simulink model "robotarm_A2_breach"  (R2018b)
settings: Solver=FixedStepAuto  StartTime=0.0  StopTime=tspan(end)  RelTol=1e-3  AbsTol=1e-6
undefined symbols (not defined in the file): options
libraries: neural x132, simulink x2
(part 2 of 6)

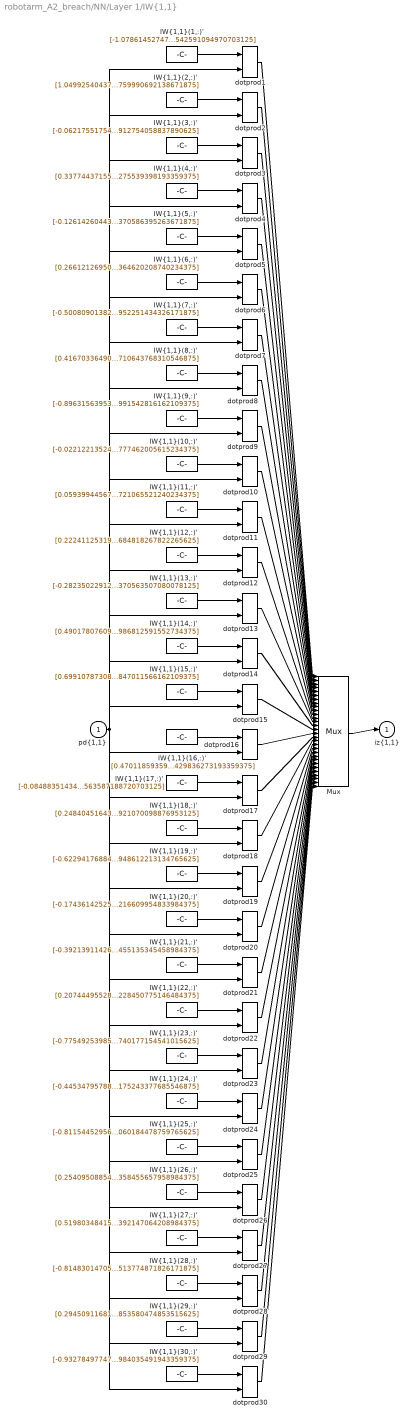
== system robotarm_A2_breach/NN/Layer 1/IW{1,1} ==
  "pd{1,1}" : Inport  PortDimensions=10
      mask Display: e = 0.06;c1 = [120 230 180]/255;c2 = ([120 230 180]+0)/(256+128);c3 = ([120 230 180]+128)/(256+128);patch([0 1 1 0],[0 0 1 1],c1);patch([0 1 1 1-e 1-e 0+e],[0 0 1 1-e 0+e 0+e],c2);patch([0 0 1 1-e 0+e 0+e],[0 1 1 1-e 1-e 0+e],c3);plot([0 1 1 0 0],[0 0 1 1 0]);
  "IW{1,1}(1,:)'" : Constant  Value=[-1.0786145274703653473835629483801312744617462158203125;0.77264081663859851545339552103541791439056396484375;0.93405870513662414555966506668482907116413116455078125;-0.012284087004165382406295492501158150844275951385498046875;-0.07882050130441907442868654243284254334867000579833984375;0.449587152172945092587497128988616168498992919921875;0.2441305252532121328190584108597249723970890045166015625;0.46267379659151774973224746645428240299224853515625;0.31528848398154940557702730075106956064701080322265625;0.592770821508250111975257823360152542591094970703125]
      mask Display: e = 0.06;c1 = [120 150 230]/255;c2 = ([120 150 230]+0)/383;c3 = ([120 150 230]+128)/383;patch([0 1 1 0],[0 0 1 1],c1);patch([0 1 1 1-e 1-e 0+e],[0 0 1 1-e 0+e 0+e],c2);patch([0 0 1 1-e 0+e 0+e],[0 1 1 1-e 1-e 0+e],c3);plot([0 1 1 0 0],[0 0 1 1 0]);disp('Weights');
  "IW{1,1}(10,:)'" : Constant  Value=[-0.02212213524676130693702447160831070505082607269287109375;0.70448840071230034443061640558880753815174102783203125;-0.38943718547013428388225975140812806785106658935546875;0.060339806407884423455900702037979499436914920806884765625;0.97898368743937858038606236732448451220989227294921875;-0.8612083675280104433369388061692006886005401611328125;0.16399922308413772409352304748608730733394622802734375;0.2354951023310313529268711363329202868044376373291015625;0.57616029420315928444296105226385407149791717529296875;-0.31121188855659320804392109494074247777462005615234375]
      mask Display: e = 0.06;c1 = [120 150 230]/255;c2 = ([120 150 230]+0)/383;c3 = ([120 150 230]+128)/383;patch([0 1 1 0],[0 0 1 1],c1);patch([0 1 1 1-e 1-e 0+e],[0 0 1 1-e 0+e 0+e],c2);patch([0 0 1 1-e 0+e 0+e],[0 1 1 1-e 1-e 0+e],c3);plot([0 1 1 0 0],[0 0 1 1 0]);disp('Weights');
  "IW{1,1}(11,:)'" : Constant  Value=[0.05939944567701915811852586557506583631038665771484375;-0.6082056891321736546984766391688026487827301025390625;1.03721893251289554171989948372356593608856201171875;0.4534212907984009888195942039601504802703857421875;-0.648457002097055035250150467618368566036224365234375;0.74638444669292958177919672380085103213787078857421875;-0.7295656890584074627525978939956985414028167724609375;0.306888274274469463609449348950874991714954376220703125;0.452997445555755662294217245289473794400691986083984375;0.62071804133911834266967844087048433721065521240234375]
      mask Display: e = 0.06;c1 = [120 150 230]/255;c2 = ([120 150 230]+0)/383;c3 = ([120 150 230]+128)/383;patch([0 1 1 0],[0 0 1 1],c1);patch([0 1 1 1-e 1-e 0+e],[0 0 1 1-e 0+e 0+e],c2);patch([0 0 1 1-e 0+e 0+e],[0 1 1 1-e 1-e 0+e],c3);plot([0 1 1 0 0],[0 0 1 1 0]);disp('Weights');
  "IW{1,1}(12,:)'" : Constant  Value=[0.2224112531983455098849589148812810890376567840576171875;0.9524124999603269525749738022568635642528533935546875;0.449678438978997230268674911712878383696079254150390625;-0.4750221129501801531347382478998042643070220947265625;-0.9211744836310391537637087822076864540576934814453125;0.052229757071233375020913314301651553250849246978759765625;0.385922954439779253288378413344617001712322235107421875;1.4936754414252713107913450585328973829746246337890625;-0.72219037687164500116665522000403143465518951416015625;0.175345525983748251608318469152436591684818267822265625]
      mask Display: e = 0.06;c1 = [120 150 230]/255;c2 = ([120 150 230]+0)/383;c3 = ([120 150 230]+128)/383;patch([0 1 1 0],[0 0 1 1],c1);patch([0 1 1 1-e 1-e 0+e],[0 0 1 1-e 0+e 0+e],c2);patch([0 0 1 1-e 0+e 0+e],[0 1 1 1-e 1-e 0+e],c3);plot([0 1 1 0 0],[0 0 1 1 0]);disp('Weights');
  "IW{1,1}(13,:)'" : Constant  Value=[-0.282350229125070517621765020521706901490688323974609375;-0.058648558215878811294974326528972596861422061920166015625;-0.57320286798997999166971339946030639111995697021484375;-0.266619245951860595056359670707024633884429931640625;0.478896997174792782292485071593546308577060699462890625;-0.75778754095938405388466208023601211607456207275390625;0.333977874970702526269406007486395537853240966796875;0.49266099516189421070322396190022118389606475830078125;-0.38191425989503702265182027986156754195690155029296875;0.43198758979670082158719424114678986370563507080078125]
      mask Display: e = 0.06;c1 = [120 150 230]/255;c2 = ([120 150 230]+0)/383;c3 = ([120 150 230]+128)/383;patch([0 1 1 0],[0 0 1 1],c1);patch([0 1 1 1-e 1-e 0+e],[0 0 1 1-e 0+e 0+e],c2);patch([0 0 1 1-e 0+e 0+e],[0 1 1 1-e 1-e 0+e],c3);plot([0 1 1 0 0],[0 0 1 1 0]);disp('Weights');
  "IW{1,1}(14,:)'" : Constant  Value=[0.490178076094217429758970183684141375124454498291015625;-0.62326983838903060597402827625046484172344207763671875;0.5009499629854321511857051518745720386505126953125;-0.816225444285765266982934917905367910861968994140625;-0.67078711304246041446930348683963529765605926513671875;0.254975206941694454432223437834181822836399078369140625;-0.278841518061437365627597273487481288611888885498046875;0.83711628486389333403394630295224487781524658203125;-0.59067831886427490939439621797646395862102508544921875;0.1565516289896598800535088003016426227986812591552734375]
      mask Display: e = 0.06;c1 = [120 150 230]/255;c2 = ([120 150 230]+0)/383;c3 = ([120 150 230]+128)/383;patch([0 1 1 0],[0 0 1 1],c1);patch([0 1 1 1-e 1-e 0+e],[0 0 1 1-e 0+e 0+e],c2);patch([0 0 1 1-e 0+e 0+e],[0 1 1 1-e 1-e 0+e],c3);plot([0 1 1 0 0],[0 0 1 1 0]);disp('Weights');
  "IW{1,1}(15,:)'" : Constant  Value=[0.69910787308807942341815078179934062063694000244140625;-0.1568376662110783914538814087791251949965953826904296875;-0.1625636975459366084795220785963465459644794464111328125;0.284408931478114135327217582016601227223873138427734375;-0.42107382523295111553807146265171468257904052734375;0.9562152907966228188030299861566163599491119384765625;0.289805319971675190426907420260249637067317962646484375;0.5149517160964600659411871674819849431514739990234375;1.050216977025737907780467139673419296741485595703125;-0.408730541549422010660919113433919847011566162109375]
      mask Display: e = 0.06;c1 = [120 150 230]/255;c2 = ([120 150 230]+0)/383;c3 = ([120 150 230]+128)/383;patch([0 1 1 0],[0 0 1 1],c1);patch([0 1 1 1-e 1-e 0+e],[0 0 1 1-e 0+e 0+e],c2);patch([0 0 1 1-e 0+e 0+e],[0 1 1 1-e 1-e 0+e],c3);plot([0 1 1 0 0],[0 0 1 1 0]);disp('Weights');
  "IW{1,1}(16,:)'" : Constant  Value=[0.4701185935926586179078867644420824944972991943359375;-0.52573176058228832108198957939748652279376983642578125;-0.51310353367696792670216154874651692807674407958984375;0.633282813875369665623793480335734784603118896484375;-0.23576962859137762240635538546484895050525665283203125;0.94962610926828083801609636793727986514568328857421875;-0.131551897207896784092184816472581587731838226318359375;-0.151782556545362268263232863318989984691143035888671875;0.63884299905071362246644639526493847370147705078125;0.92640223794052045658276028916588984429836273193359375]
      mask Display: e = 0.06;c1 = [120 150 230]/255;c2 = ([120 150 230]+0)/383;c3 = ([120 150 230]+128)/383;patch([0 1 1 0],[0 0 1 1],c1);patch([0 1 1 1-e 1-e 0+e],[0 0 1 1-e 0+e 0+e],c2);patch([0 0 1 1-e 0+e 0+e],[0 1 1 1-e 1-e 0+e],c3);plot([0 1 1 0 0],[0 0 1 1 0]);disp('Weights');
  "IW{1,1}(17,:)'" : Constant  Value=[-0.08488351434668546524608956360680167563259601593017578125;-0.1776452243687499932267570557087310589849948883056640625;0.51172192885572076459510526547092013061046600341796875;0.04987808261153768574214240061337477527558803558349609375;-0.43208410477753600442696324535063467919826507568359375;-0.18514863404363401944152656142250634729862213134765625;0.8180515394720269117811994874500669538974761962890625;-0.404768665009769323948063401985564269125461578369140625;-0.78330152213928816440358104955521412193775177001953125;1.2056407408852092277840029055369086563587188720703125]
      mask Display: e = 0.06;c1 = [120 150 230]/255;c2 = ([120 150 230]+0)/383;c3 = ([120 150 230]+128)/383;patch([0 1 1 0],[0 0 1 1],c1);patch([0 1 1 1-e 1-e 0+e],[0 0 1 1-e 0+e 0+e],c2);patch([0 0 1 1-e 0+e 0+e],[0 1 1 1-e 1-e 0+e],c3);plot([0 1 1 0 0],[0 0 1 1 0]);disp('Weights');
  "IW{1,1}(18,:)'" : Constant  Value=[0.2484045164372511715900060380590730346739292144775390625;-0.57530685825965599544673523269011639058589935302734375;0.60142104775230909030625525701907463371753692626953125;0.226128051472227864504560557179502211511135101318359375;-0.630503249581572777771043547545559704303741455078125;-0.7272929920174118212372604830306954681873321533203125;0.11569360803807045290358956890486297197639942169189453125;-0.67078212474529663733591178242932073771953582763671875;-0.67017373266770141615467082374379970133304595947265625;0.48396773279367100162318138245609588921070098876953125]
      mask Display: e = 0.06;c1 = [120 150 230]/255;c2 = ([120 150 230]+0)/383;c3 = ([120 150 230]+128)/383;patch([0 1 1 0],[0 0 1 1],c1);patch([0 1 1 1-e 1-e 0+e],[0 0 1 1-e 0+e 0+e],c2);patch([0 0 1 1-e 0+e 0+e],[0 1 1 1-e 1-e 0+e],c3);plot([0 1 1 0 0],[0 0 1 1 0]);disp('Weights');
  "IW{1,1}(19,:)'" : Constant  Value=[-0.62294176884013030548459255442139692604541778564453125;1.228614141570630646782547046313993632793426513671875;-0.65153079809169101022092718267231248319149017333984375;-0.17866952508290323553552525481791235506534576416015625;0.40869256223672090211351815014495514333248138427734375;-0.12746962924570592878836805539322085678577423095703125;0.79148363856496850576860424553160555660724639892578125;-0.201395605907412733603933929771301336586475372314453125;0.1093193723382310522662663743176381103694438934326171875;0.250553370603376512892879190985695458948612213134765625]
      mask Display: e = 0.06;c1 = [120 150 230]/255;c2 = ([120 150 230]+0)/383;c3 = ([120 150 230]+128)/383;patch([0 1 1 0],[0 0 1 1],c1);patch([0 1 1 1-e 1-e 0+e],[0 0 1 1-e 0+e 0+e],c2);patch([0 0 1 1-e 0+e 0+e],[0 1 1 1-e 1-e 0+e],c3);plot([0 1 1 0 0],[0 0 1 1 0]);disp('Weights');
  "IW{1,1}(2,:)'" : Constant  Value=[1.0499254043761692134495433492702431976795196533203125;0.61799414227169735536193684311001561582088470458984375;-0.52447623404908194633122775485389865934848785400390625;-0.287937489300537918790467983853886835277080535888671875;0.1344168212775924964308416065250639803707599639892578125;-0.05313191843903837530138645206534420140087604522705078125;0.6158784457077006724290413330891169607639312744140625;-0.0245661774092495177601591649363399483263492584228515625;0.6310651001964746598105193697847425937652587890625;0.78336995872014625330592707541654817759990692138671875]
      mask Display: e = 0.06;c1 = [120 150 230]/255;c2 = ([120 150 230]+0)/383;c3 = ([120 150 230]+128)/383;patch([0 1 1 0],[0 0 1 1],c1);patch([0 1 1 1-e 1-e 0+e],[0 0 1 1-e 0+e 0+e],c2);patch([0 0 1 1-e 0+e 0+e],[0 1 1 1-e 1-e 0+e],c3);plot([0 1 1 0 0],[0 0 1 1 0]);disp('Weights');
  "IW{1,1}(20,:)'" : Constant  Value=[-0.1743614252579658019381980693651712499558925628662109375;0.17949361845256817105109803378582000732421875;-0.9601260579391561744699856717488728463649749755859375;0.8936497347696434889741112783667631447315216064453125;0.1001117015390539377595047199065447784960269927978515625;-0.224771645110486473218003311558277346193790435791015625;-0.390238429406900733109608836457482539117336273193359375;-0.11534957973063413028125268056101049296557903289794921875;-1.0076789430020338667048918068758212029933929443359375;-0.27983387043521845694016292327432893216609954833984375]
      mask Display: e = 0.06;c1 = [120 150 230]/255;c2 = ([120 150 230]+0)/383;c3 = ([120 150 230]+128)/383;patch([0 1 1 0],[0 0 1 1],c1);patch([0 1 1 1-e 1-e 0+e],[0 0 1 1-e 0+e 0+e],c2);patch([0 0 1 1-e 0+e 0+e],[0 1 1 1-e 1-e 0+e],c3);plot([0 1 1 0 0],[0 0 1 1 0]);disp('Weights');
  "IW{1,1}(21,:)'" : Constant  Value=[-0.392139114269041078042477010967559181153774261474609375;-0.6199488458763384723937406306504271924495697021484375;-0.63464659170326898074421251294552348554134368896484375;0.99833692946451091376758313344907946884632110595703125;0.002249719025076850169309050642141301068477332592010498046875;-0.90000854269888963532508796561160124838352203369140625;0.06136728531872741310149166338305803947150707244873046875;-0.058406780188430762468243528928724117577075958251953125;0.75847883298217599890023166153696365654468536376953125;0.41485044328498987820097454459755681455135345458984375]
      mask Display: e = 0.06;c1 = [120 150 230]/255;c2 = ([120 150 230]+0)/383;c3 = ([120 150 230]+128)/383;patch([0 1 1 0],[0 0 1 1],c1);patch([0 1 1 1-e 1-e 0+e],[0 0 1 1-e 0+e 0+e],c2);patch([0 0 1 1-e 0+e 0+e],[0 1 1 1-e 1-e 0+e],c3);plot([0 1 1 0 0],[0 0 1 1 0]);disp('Weights');
  "IW{1,1}(22,:)'" : Constant  Value=[0.207444955287041654656832179171033203601837158203125;-1.0115942500225398870128401540569029748439788818359375;-0.08263739871460083763476944795911549590528011322021484375;0.19625568705457607787678853128454647958278656005859375;0.0549960717494557826956480539593030698597431182861328125;1.07069693218174766258243835181929171085357666015625;-0.82673959179818024001207277251523919403553009033203125;-0.206721188223280283313698646452394314110279083251953125;-0.323782228784486869610503845251514576375484466552734375;0.82513657952248864457800436866818927228450775146484375]
      mask Display: e = 0.06;c1 = [120 150 230]/255;c2 = ([120 150 230]+0)/383;c3 = ([120 150 230]+128)/383;patch([0 1 1 0],[0 0 1 1],c1);patch([0 1 1 1-e 1-e 0+e],[0 0 1 1-e 0+e 0+e],c2);patch([0 0 1 1-e 0+e 0+e],[0 1 1 1-e 1-e 0+e],c3);plot([0 1 1 0 0],[0 0 1 1 0]);disp('Weights');
  "IW{1,1}(23,:)'" : Constant  Value=[-0.77549253985802046873487824996118433773517608642578125;0.82504860349101161176577079459093511104583740234375;0.8627943940992668370171259084600023925304412841796875;0.049177727324097537942027003055045497603714466094970703125;0.272756037877112278433600067728548310697078704833984375;-0.3944377653609512091037458958453498780727386474609375;-0.278065662283786652064776490078656934201717376708984375;-0.85084809478306866470376235156436450779438018798828125;-0.2392235789523589895022581686134799383580684661865234375;-0.11726281585353660885662208102075965143740177154541015625]
      mask Display: e = 0.06;c1 = [120 150 230]/255;c2 = ([120 150 230]+0)/383;c3 = ([120 150 230]+128)/383;patch([0 1 1 0],[0 0 1 1],c1);patch([0 1 1 1-e 1-e 0+e],[0 0 1 1-e 0+e 0+e],c2);patch([0 0 1 1-e 0+e 0+e],[0 1 1 1-e 1-e 0+e],c3);plot([0 1 1 0 0],[0 0 1 1 0]);disp('Weights');
  "IW{1,1}(24,:)'" : Constant  Value=[-0.445347957881927547507672215942875482141971588134765625;1.0809176259228205907447772915475070476531982421875;-0.40201497015928067124690414857468567788600921630859375;-0.39139803547385965121208073469460941851139068603515625;-0.5122521596410261057741308832191862165927886962890625;1.3112835772537534406723125357530079782009124755859375;0.41453577108138350837407415383495390415191650390625;-0.303522385230105218312246506684459745883941650390625;0.1373937183372464232444798426513443700969219207763671875;0.1989843605931122805241528794795158319175243377685546875]
      mask Display: e = 0.06;c1 = [120 150 230]/255;c2 = ([120 150 230]+0)/383;c3 = ([120 150 230]+128)/383;patch([0 1 1 0],[0 0 1 1],c1);patch([0 1 1 1-e 1-e 0+e],[0 0 1 1-e 0+e 0+e],c2);patch([0 0 1 1-e 0+e 0+e],[0 1 1 1-e 1-e 0+e],c3);plot([0 1 1 0 0],[0 0 1 1 0]);disp('Weights');
  "IW{1,1}(25,:)'" : Constant  Value=[-0.8115445295642180756345851477817632257938385009765625;0.85652359166349312236121704700053669512271881103515625;-0.040112309950283531190251551379333250224590301513671875;0.34139068256503424247938482949393801391124725341796875;-0.0165130756249407158187114674774420564062893390655517578125;0.1727717610732415476348933225381188094615936279296875;-0.56275702056715581900192546527250669896602630615234375;-0.469766238140822578461808234351337887346744537353515625;-0.7689193778683238722493342720554210245609283447265625;0.43278481301085369725711871069506742060184478759765625]
      mask Display: e = 0.06;c1 = [120 150 230]/255;c2 = ([120 150 230]+0)/383;c3 = ([120 150 230]+128)/383;patch([0 1 1 0],[0 0 1 1],c1);patch([0 1 1 1-e 1-e 0+e],[0 0 1 1-e 0+e 0+e],c2);patch([0 0 1 1-e 0+e 0+e],[0 1 1 1-e 1-e 0+e],c3);plot([0 1 1 0 0],[0 0 1 1 0]);disp('Weights');
  "IW{1,1}(26,:)'" : Constant  Value=[0.254095088548551839569000776464235968887805938720703125;0.5486404111308582631778563154512085020542144775390625;0.5622493049893790839632856659591197967529296875;0.174248576368332852570830482363817282021045684814453125;-1.166774243979380454305783132440410554409027099609375;-0.413594460099152072540817925982992164790630340576171875;0.30982398051400716898484688499593175947666168212890625;-0.2248549620127749670839278905987157486379146575927734375;0.1834613666491745342934649443122907541692256927490234375;-0.81852663874897702012134459437220357358455657958984375]
      mask Display: e = 0.06;c1 = [120 150 230]/255;c2 = ([120 150 230]+0)/383;c3 = ([120 150 230]+128)/383;patch([0 1 1 0],[0 0 1 1],c1);patch([0 1 1 1-e 1-e 0+e],[0 0 1 1-e 0+e 0+e],c2);patch([0 0 1 1-e 0+e 0+e],[0 1 1 1-e 1-e 0+e],c3);plot([0 1 1 0 0],[0 0 1 1 0]);disp('Weights');
  "IW{1,1}(27,:)'" : Constant  Value=[0.519803484154455208710032820818014442920684814453125;-0.98664054697819725259222423119354061782360076904296875;0.8322529575162087578377168028964661061763763427734375;-0.21234182155734970809390915746917016804218292236328125;-0.625224818042553476260536626796238124370574951171875;-0.418449264732979331338214024071930907666683197021484375;0.5003880606650217277575620755669660866260528564453125;-0.47645348059044601018996445418451912701129913330078125;-0.83071497620484813229069231965695507824420928955078125;-0.332557223531743717526154568986385129392147064208984375]
      mask Display: e = 0.06;c1 = [120 150 230]/255;c2 = ([120 150 230]+0)/383;c3 = ([120 150 230]+128)/383;patch([0 1 1 0],[0 0 1 1],c1);patch([0 1 1 1-e 1-e 0+e],[0 0 1 1-e 0+e 0+e],c2);patch([0 0 1 1-e 0+e 0+e],[0 1 1 1-e 1-e 0+e],c3);plot([0 1 1 0 0],[0 0 1 1 0]);disp('Weights');
  "IW{1,1}(28,:)'" : Constant  Value=[-0.814830147056870401911510271020233631134033203125;0.64023075046793243014775498522794805467128753662109375;0.07998590248178626127550927549236803315579891204833984375;0.7468624036618856099067897957866080105304718017578125;-1.1056137600491295902571664555580355226993560791015625;0.430918947841503807705265671756933443248271942138671875;-0.558748606104922718174066176288761198520660400390625;0.104602745800456309321901926523423753678798675537109375;0.413069878341958851564186261384747922420501708984375;0.75799997126023199722766321428935043513774871826171875]
      mask Display: e = 0.06;c1 = [120 150 230]/255;c2 = ([120 150 230]+0)/383;c3 = ([120 150 230]+128)/383;patch([0 1 1 0],[0 0 1 1],c1);patch([0 1 1 1-e 1-e 0+e],[0 0 1 1-e 0+e 0+e],c2);patch([0 0 1 1-e 0+e 0+e],[0 1 1 1-e 1-e 0+e],c3);plot([0 1 1 0 0],[0 0 1 1 0]);disp('Weights');
  "IW{1,1}(29,:)'" : Constant  Value=[0.29450911681218705506779542702133767306804656982421875;0.749004580041173984028546328772790729999542236328125;-0.1570668618363682822458571308743557892739772796630859375;-0.8398685428363703575627141617587767541408538818359375;-0.6081768114887093901188563904725015163421630859375;0.32478499611193722973467856718343682587146759033203125;0.286771973765567123049180509042344056069850921630859375;-0.03238632895771877129309501697207451798021793365478515625;-1.0254886670478768895264920502086170017719268798828125;-0.2471036802149940980743991758572519756853580474853515625]
      mask Display: e = 0.06;c1 = [120 150 230]/255;c2 = ([120 150 230]+0)/383;c3 = ([120 150 230]+128)/383;patch([0 1 1 0],[0 0 1 1],c1);patch([0 1 1 1-e 1-e 0+e],[0 0 1 1-e 0+e 0+e],c2);patch([0 0 1 1-e 0+e 0+e],[0 1 1 1-e 1-e 0+e],c3);plot([0 1 1 0 0],[0 0 1 1 0]);disp('Weights');
  "IW{1,1}(3,:)'" : Constant  Value=[-0.062175517549275693962584909968427382409572601318359375;0.79976020189601459975392572232522070407867431640625;0.802914082800883388557622311054728925228118896484375;-0.690380306074979355202003716840408742427825927734375;-0.048837903690828500524734323562370263971388339996337890625;0.11029200924232045177841854410871746949851512908935546875;0.91587780721977607445438707145513035356998443603515625;-0.91066893873616916454949432591092772781848907470703125;0.670390402897874881915640798979438841342926025390625;0.1290439500641699377414539640085422433912754058837890625]
      mask Display: e = 0.06;c1 = [120 150 230]/255;c2 = ([120 150 230]+0)/383;c3 = ([120 150 230]+128)/383;patch([0 1 1 0],[0 0 1 1],c1);patch([0 1 1 1-e 1-e 0+e],[0 0 1 1-e 0+e 0+e],c2);patch([0 0 1 1-e 0+e 0+e],[0 1 1 1-e 1-e 0+e],c3);plot([0 1 1 0 0],[0 0 1 1 0]);disp('Weights');
  "IW{1,1}(30,:)'" : Constant  Value=[-0.93278497747409561124953825128613971173763275146484375;0.042750716319125865727546198513664421625435352325439453125;-0.382519205900573033840572634289856068789958953857421875;0.268643851815698886387195898350910283625125885009765625;0.09135765957295725880893400017157546244561672210693359375;0.3447290892171170906266297606634907424449920654296875;0.729785766409233982443538479856215417385101318359375;0.1525900523669900532564014383751782588660717010498046875;-0.463703090881194823769106960753560997545719146728515625;-0.6957300273642257337769478908739984035491943359375]
      mask Display: e = 0.06;c1 = [120 150 230]/255;c2 = ([120 150 230]+0)/383;c3 = ([120 150 230]+128)/383;patch([0 1 1 0],[0 0 1 1],c1);patch([0 1 1 1-e 1-e 0+e],[0 0 1 1-e 0+e 0+e],c2);patch([0 0 1 1-e 0+e 0+e],[0 1 1 1-e 1-e 0+e],c3);plot([0 1 1 0 0],[0 0 1 1 0]);disp('Weights');
  "IW{1,1}(4,:)'" : Constant  Value=[0.337744371552312905304660262117977254092693328857421875;0.438658492688066392606316412638989277184009552001953125;0.346762484572657292414277208081330172717571258544921875;0.01462330612340994630271584497904768795706331729888916015625;0.0983481465700370149907172390157938934862613677978515625;0.464560857145485617269997646872070617973804473876953125;1.01070810266281174705227385857142508029937744140625;-0.87382707478694221503445760390604846179485321044921875;1.0496441423824671712594636119320057332515716552734375;0.0248224303270956590805607078209504834376275539398193359375]
      mask Display: e = 0.06;c1 = [120 150 230]/255;c2 = ([120 150 230]+0)/383;c3 = ([120 150 230]+128)/383;patch([0 1 1 0],[0 0 1 1],c1);patch([0 1 1 1-e 1-e 0+e],[0 0 1 1-e 0+e 0+e],c2);patch([0 0 1 1-e 0+e 0+e],[0 1 1 1-e 1-e 0+e],c3);plot([0 1 1 0 0],[0 0 1 1 0]);disp('Weights');
  "IW{1,1}(5,:)'" : Constant  Value=[-0.1261426044360567655377991513887536711990833282470703125;1.085407332502960731090979606960900127887725830078125;-0.6093806028663932838895789245725609362125396728515625;0.47052339319611846679691780082066543400287628173828125;-1.2781125217893827272774842640501447021961212158203125;0.17527458377895965835335800875327549874782562255859375;-0.163833123110417477885647485891240648925304412841796875;0.57965330683325344551803937065415084362030029296875;0.42939310245523254483401842662715353071689605712890625;0.175284925303460681345057992075453512370586395263671875]
      mask Display: e = 0.06;c1 = [120 150 230]/255;c2 = ([120 150 230]+0)/383;c3 = ([120 150 230]+128)/383;patch([0 1 1 0],[0 0 1 1],c1);patch([0 1 1 1-e 1-e 0+e],[0 0 1 1-e 0+e 0+e],c2);patch([0 0 1 1-e 0+e 0+e],[0 1 1 1-e 1-e 0+e],c3);plot([0 1 1 0 0],[0 0 1 1 0]);disp('Weights');
  "IW{1,1}(6,:)'" : Constant  Value=[0.266121269504327795374365450697951018810272216796875;0.345289957695091132006126599662820808589458465576171875;-0.405324426484343913745789222957682795822620391845703125;-0.75194254661663151306782992833177559077739715576171875;-0.37360942358920812278455514388042502105236053466796875;-0.75453090073678785731914331336156465113162994384765625;0.0218035224725904031028989038532017730176448822021484375;0.94226287381246531804634969375911168754100799560546875;0.78737097953365331459707476824405603110790252685546875;-0.401068310039879472039814345407648943364620208740234375]
      mask Display: e = 0.06;c1 = [120 150 230]/255;c2 = ([120 150 230]+0)/383;c3 = ([120 150 230]+128)/383;patch([0 1 1 0],[0 0 1 1],c1);patch([0 1 1 1-e 1-e 0+e],[0 0 1 1-e 0+e 0+e],c2);patch([0 0 1 1-e 0+e 0+e],[0 1 1 1-e 1-e 0+e],c3);plot([0 1 1 0 0],[0 0 1 1 0]);disp('Weights');
  "IW{1,1}(7,:)'" : Constant  Value=[-0.5008090138215361974971528979949653148651123046875;1.2758507874578068896909144314122386276721954345703125;0.382550490429632350508626359442132525146007537841796875;-0.47586297800645283029297161192516796290874481201171875;0.07887070455056723050635270055863657034933567047119140625;-0.87628661722909428899441763860522769391536712646484375;0.52707567806589106229608887588256038725376129150390625;-0.55337939883954512243491308254306204617023468017578125;-0.165740253572662477044019624372594989836215972900390625;-0.53762987932637329446805551924626342952251434326171875]
      mask Display: e = 0.06;c1 = [120 150 230]/255;c2 = ([120 150 230]+0)/383;c3 = ([120 150 230]+128)/383;patch([0 1 1 0],[0 0 1 1],c1);patch([0 1 1 1-e 1-e 0+e],[0 0 1 1-e 0+e 0+e],c2);patch([0 0 1 1-e 0+e 0+e],[0 1 1 1-e 1-e 0+e],c3);plot([0 1 1 0 0],[0 0 1 1 0]);disp('Weights');
  "IW{1,1}(8,:)'" : Constant  Value=[0.416703364907324125265830616626772098243236541748046875;-0.95208511548533325541399108260520733892917633056640625;0.64051919526938483340217089789803139865398406982421875;0.03566479432376194746989739314813050441443920135498046875;-0.450653349711516104658670656135655008256435394287109375;1.313122279786888224606400399352423846721649169921875;-0.632412010736363328078368795104324817657470703125;-0.1444743209525030380735444168749381788074970245361328125;0.4332492700076944203146922518499195575714111328125;0.94903664465549109063857713408651761710643768310546875]
      mask Display: e = 0.06;c1 = [120 150 230]/255;c2 = ([120 150 230]+0)/383;c3 = ([120 150 230]+128)/383;patch([0 1 1 0],[0 0 1 1],c1);patch([0 1 1 1-e 1-e 0+e],[0 0 1 1-e 0+e 0+e],c2);patch([0 0 1 1-e 0+e 0+e],[0 1 1 1-e 1-e 0+e],c3);plot([0 1 1 0 0],[0 0 1 1 0]);disp('Weights');
  "IW{1,1}(9,:)'" : Constant  Value=[-0.896315639538358244209348413278348743915557861328125;0.92860680590292854486023088611545972526073455810546875;-0.35755386459640170482288112907554022967815399169921875;0.58532610555969366572526269010268151760101318359375;-0.2198462310062675728605796621195622719824314117431640625;0.2415783437075041673036679412689409218728542327880859375;-0.26631578004203826370854812921606935560703277587890625;0.286716388232604757480004309400101192295551300048828125;0.6334605630026761691198089465615339577198028564453125;-0.055683207954953982399270984160466468892991542816162109375]
      mask Display: e = 0.06;c1 = [120 150 230]/255;c2 = ([120 150 230]+0)/383;c3 = ([120 150 230]+128)/383;patch([0 1 1 0],[0 0 1 1],c1);patch([0 1 1 1-e 1-e 0+e],[0 0 1 1-e 0+e 0+e],c2);patch([0 0 1 1-e 0+e 0+e],[0 1 1 1-e 1-e 0+e],c3);plot([0 1 1 0 0],[0 0 1 1 0]);disp('Weights');
  Mux : Mux  Inputs=30
      mask Display: e = 0.06;c1 = [120 150 230]/255;c2 = ([120 150 230]+0)/383;c3 = ([120 150 230]+128)/383;patch([0 1 1 0],[0 0 1 1],c1);patch([0 1 1 1-e 1-e 0+e],[0 0 1 1-e 0+e 0+e],c2);patch([0 0 1 1-e 0+e 0+e],[0 1 1 1-e 1-e 0+e],c3);plot([0 1 1 0 0],[0 0 1 1 0]);disp('Mux');
  dotprod{1..30} (30 alike) : neural/Weight Functions/dotprod
  "iz{1,1}" : Outport
      mask Display: e = 0.06;c1 = [120 230 180]/255;c2 = ([120 230 180]+0)/(256+128);c3 = ([120 230 180]+128)/(256+128);patch([0 1 1 0],[0 0 1 1],c1);patch([0 1 1 1-e 1-e 0+e],[0 0 1 1-e 0+e 0+e],c2);patch([0 0 1 1-e 0+e 0+e],[0 1 1 1-e 1-e 0+e],c3);plot([0 1 1 0 0],[0 0 1 1 0]);
  wires:
  "IW{1,1}(1,:)'"/1 -> dotprod1/1
  "pd{1,1}"/1 -> dotprod1/2, dotprod2/2, dotprod3/2, dotprod4/2, dotprod5/2, dotprod6/2, dotprod7/2, dotprod8/2, dotprod9/2, dotprod10/2, dotprod11/2, dotprod12/2, dotprod13/2, dotprod14/2, dotprod15/2, dotprod16/2, dotprod17/2, dotprod18/2, dotprod19/2, dotprod20/2, dotprod21/2, dotprod22/2, dotprod23/2, dotprod24/2, dotprod25/2, dotprod26/2, dotprod27/2, dotprod28/2, dotprod29/2, dotprod30/2
  dotprod1/1 -> Mux/1
  "IW{1,1}(2,:)'"/1 -> dotprod2/1
  dotprod2/1 -> Mux/2
  "IW{1,1}(3,:)'"/1 -> dotprod3/1
  dotprod3/1 -> Mux/3
  "IW{1,1}(4,:)'"/1 -> dotprod4/1
  dotprod4/1 -> Mux/4
  "IW{1,1}(5,:)'"/1 -> dotprod5/1
  dotprod5/1 -> Mux/5
  "IW{1,1}(6,:)'"/1 -> dotprod6/1
  dotprod6/1 -> Mux/6
  "IW{1,1}(7,:)'"/1 -> dotprod7/1
  dotprod7/1 -> Mux/7
  "IW{1,1}(8,:)'"/1 -> dotprod8/1
  dotprod8/1 -> Mux/8
  "IW{1,1}(9,:)'"/1 -> dotprod9/1
  dotprod9/1 -> Mux/9
  "IW{1,1}(10,:)'"/1 -> dotprod10/1
  dotprod10/1 -> Mux/10
  "IW{1,1}(11,:)'"/1 -> dotprod11/1
  dotprod11/1 -> Mux/11
  "IW{1,1}(12,:)'"/1 -> dotprod12/1
  dotprod12/1 -> Mux/12
  "IW{1,1}(13,:)'"/1 -> dotprod13/1
  dotprod13/1 -> Mux/13
  "IW{1,1}(14,:)'"/1 -> dotprod14/1
  dotprod14/1 -> Mux/14
  "IW{1,1}(15,:)'"/1 -> dotprod15/1
  dotprod15/1 -> Mux/15
  "IW{1,1}(16,:)'"/1 -> dotprod16/1
  dotprod16/1 -> Mux/16
  "IW{1,1}(17,:)'"/1 -> dotprod17/1
  dotprod17/1 -> Mux/17
  "IW{1,1}(18,:)'"/1 -> dotprod18/1
  dotprod18/1 -> Mux/18
  "IW{1,1}(19,:)'"/1 -> dotprod19/1
  dotprod19/1 -> Mux/19
  "IW{1,1}(20,:)'"/1 -> dotprod20/1
  dotprod20/1 -> Mux/20
  "IW{1,1}(21,:)'"/1 -> dotprod21/1
  dotprod21/1 -> Mux/21
  "IW{1,1}(22,:)'"/1 -> dotprod22/1
  dotprod22/1 -> Mux/22
  "IW{1,1}(23,:)'"/1 -> dotprod23/1
  dotprod23/1 -> Mux/23
  "IW{1,1}(24,:)'"/1 -> dotprod24/1
  dotprod24/1 -> Mux/24
  "IW{1,1}(25,:)'"/1 -> dotprod25/1
  dotprod25/1 -> Mux/25
  "IW{1,1}(26,:)'"/1 -> dotprod26/1
  dotprod26/1 -> Mux/26
  "IW{1,1}(27,:)'"/1 -> dotprod27/1
  dotprod27/1 -> Mux/27
  "IW{1,1}(28,:)'"/1 -> dotprod28/1
  dotprod28/1 -> Mux/28
  "IW{1,1}(29,:)'"/1 -> dotprod29/1
  dotprod29/1 -> Mux/29
  "IW{1,1}(30,:)'"/1 -> dotprod30/1
  dotprod30/1 -> Mux/30
  Mux/1 -> "iz{1,1}"/1

== system robotarm_A2_breach/NN/Layer 2/Delays 1 ==
  "p{2}" : Inport  PortDimensions=30
      mask Display: e = 0.06;c1 = [120 230 180]/255;c2 = ([120 230 180]+0)/(256+128);c3 = ([120 230 180]+128)/(256+128);patch([0 1 1 0],[0 0 1 1],c1);patch([0 1 1 1-e 1-e 0+e],[0 0 1 1-e 0+e 0+e],c2);patch([0 0 1 1-e 0+e 0+e],[0 1 1 1-e 1-e 0+e],c3);plot([0 1 1 0 0],[0 0 1 1 0]);
  mux : Mux  Inputs=1
      mask Display: e = 0.06;c1 = [120 150 230]/255;c2 = ([120 150 230]+0)/383;c3 = ([120 150 230]+128)/383;patch([0 1 1 0],[0 0 1 1],c1);patch([0 1 1 1-e 1-e 0+e],[0 0 1 1-e 0+e 0+e],c2);patch([0 0 1 1-e 0+e 0+e],[0 1 1 1-e 1-e 0+e],c3);plot([0 1 1 0 0],[0 0 1 1 0]);disp('Mux')
  "pd{2,1}" : Outport
      mask Display: e = 0.06;c1 = [120 230 180]/255;c2 = ([120 230 180]+0)/(256+128);c3 = ([120 230 180]+128)/(256+128);patch([0 1 1 0],[0 0 1 1],c1);patch([0 1 1 1-e 1-e 0+e],[0 0 1 1-e 0+e 0+e],c2);patch([0 0 1 1-e 0+e 0+e],[0 1 1 1-e 1-e 0+e],c3);plot([0 1 1 0 0],[0 0 1 1 0]);
  wires:
  "p{2}"/1 -> mux/1
  mux/1 -> "pd{2,1}"/1
